simulink model "planarModel"  (R2018b)
settings: Solver=FixedStepAuto  StartTime=0.0  StopTime=50  FixedStep=0.025  RelTol=1e-3
InitFcn:
  | loadThrusterData
settings Model: Creator=Andy  LastModifiedBy=barthal
settings ModelReferenceCC: ModelReferenceNumInstancesAllowed=Single
settings RTWCC: GenCodeOnly=on

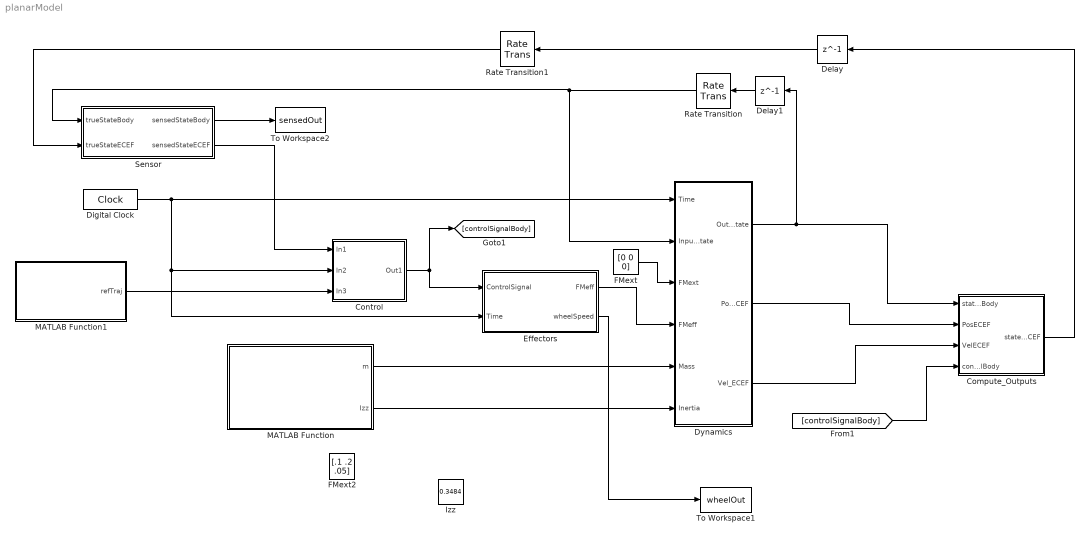
== system planarModel ==
  Compute_Outputs : Subsystem
  Control : Subsystem
  Delay : Delay  DelayLength=1
  Delay1 : Delay  DelayLength=1
  Digital Clock : DigitalClock  SampleTime=0.025
  Dynamics : Subsystem  TreatAsAtomicUnit=on
      settings: MinAlgLoopOccurrences=on
  Effectors : Subsystem  TreatAsAtomicUnit=on
  FMext : Constant  Value=[0 0 0]
  FMext2 : Constant  Value=[.1 .2 .05]
  Izz : Constant  Value=0.3484
  MATLAB Function : MATLAB Function  TreatAsAtomicUnit=on
  MATLAB Function1 : MATLAB Function  TreatAsAtomicUnit=on
  Rate Transition : RateTransition  InitialCondition=[0 0 0 0 0 0 0 0 0]
  Rate Transition1 : RateTransition  InitialCondition=[0 0 0 0 0 0 0 0 0]
  Sensor : Subsystem
  To Workspace1 : ToWorkspace  VariableName=wheelOut  SaveFormat=Timeseries  SampleTime=-1
  To Workspace2 : ToWorkspace  VariableName=sensedOut  SaveFormat=Timeseries  SampleTime=-1
  wires:
  Digital Clock/1 -> Dynamics/1(Time), Control/2(In2), Effectors/2(Time)
  FMext/1 -> Dynamics/3(FMext)
  MATLAB Function/1(m) -> Dynamics/5(Mass)
  Effectors/2(wheelSpeed) -> To Workspace1/1
  Control/1(Out1) -> [controlSignalBody], Effectors/1(ControlSignal)
  Effectors/1(FMeff) -> Dynamics/4(FMeff)
  Dynamics/1(OutputState) -> Delay1/1, Compute_Outputs/1(stateInBody)
  Dynamics/2(Pos_ECEF) -> Compute_Outputs/2(PosECEF)
  Dynamics/3(Vel_ECEF) -> Compute_Outputs/3(VelECEF)
  Compute_Outputs/1(stateOutECEF) -> Delay/1
  [controlSignalBody] -> Compute_Outputs/4(controlSignalBody)
  MATLAB Function/2(Izz) -> Dynamics/6(Inertia)
  Rate Transition/1 -> Sensor/1(trueStateBody), Dynamics/2(InputState)
  Rate Transition1/1 -> Sensor/2(trueStateECEF)
  Sensor/2(sensedStateECEF) -> Control/1(In1)
  Sensor/1(sensedStateBody) -> To Workspace2/1
  MATLAB Function1/1(refTraj) -> Control/3(In3)
  Delay/1 -> Rate Transition1/1
  Delay1/1 -> Rate Transition/1

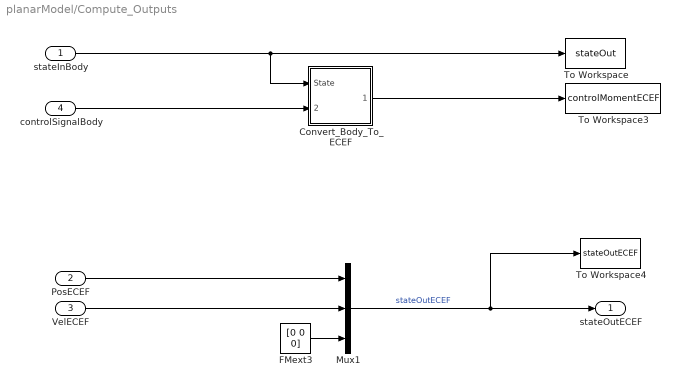
== system planarModel/Compute_Outputs ==
  stateInBody : Inport
  PosECEF : Inport  Port=2
  VelECEF : Inport  Port=3
  controlSignalBody : Inport  Port=4
  Convert_Body_To_ECEF : Subsystem
  FMext3 : Constant  Value=[0 0 0]
  Mux1 : Mux  Inputs=3
  To Workspace : ToWorkspace  VariableName=stateOut  SaveFormat=Timeseries  SampleTime=-1
  To Workspace3 : ToWorkspace  VariableName=controlMomentECEF  SaveFormat=Timeseries  SampleTime=-1
  To Workspace4 : ToWorkspace  VariableName=stateOutECEF  SaveFormat=Timeseries  SampleTime=-1
  stateOutECEF : Outport
  wires:
  Mux1/1 -> stateOutECEF/1, To Workspace4/1  "stateOutECEF"
  FMext3/1 -> Mux1/3
  stateInBody/1 -> Convert_Body_To_ECEF/1(State), To Workspace/1
  Convert_Body_To_ECEF/1(Vec_ECEF) -> To Workspace3/1
  controlSignalBody/1 -> Convert_Body_To_ECEF/2(Vec_Body)
  PosECEF/1 -> Mux1/1
  VelECEF/1 -> Mux1/2

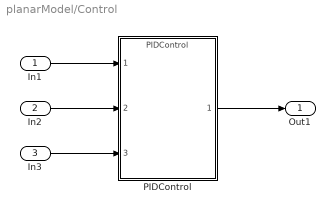
== system planarModel/Control ==
  In1 : Inport
  In2 : Inport  Port=2
  In3 : Inport  Port=3
  PIDControl : ModelReference  ModelNameDialog=PIDControl  SimulationMode=Normal  ModelReferenceVersion=1.303
  Out1 : Outport
  wires:
  In3/1 -> PIDControl/3
  In2/1 -> PIDControl/2
  PIDControl/1 -> Out1/1
  In1/1 -> PIDControl/1

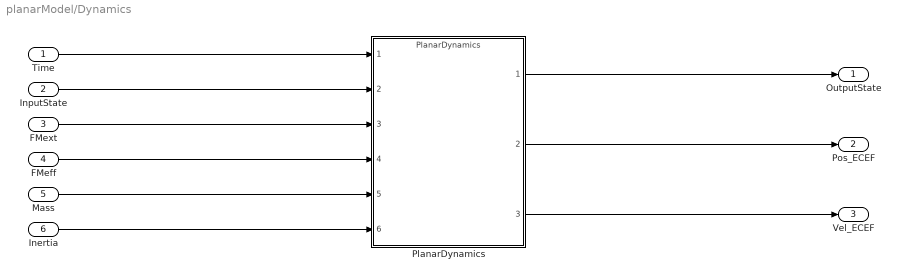
== system planarModel/Dynamics ==
  Time : Inport
  InputState : Inport  Port=2
  FMext : Inport  Port=3
  FMeff : Inport  Port=4
  Mass : Inport  Port=5
  Inertia : Inport  Port=6
  PlanarDynamics : ModelReference  ModelNameDialog=PlanarDynamics  SimulationMode=Normal  ModelReferenceVersion=1.307
  OutputState : Outport
  Pos_ECEF : Outport  Port=2
  Vel_ECEF : Outport  Port=3
  wires:
  Time/1 -> PlanarDynamics/1
  InputState/1 -> PlanarDynamics/2
  FMext/1 -> PlanarDynamics/3
  FMeff/1 -> PlanarDynamics/4
  Mass/1 -> PlanarDynamics/5
  Inertia/1 -> PlanarDynamics/6
  PlanarDynamics/1 -> OutputState/1
  PlanarDynamics/2 -> Pos_ECEF/1
  PlanarDynamics/3 -> Vel_ECEF/1

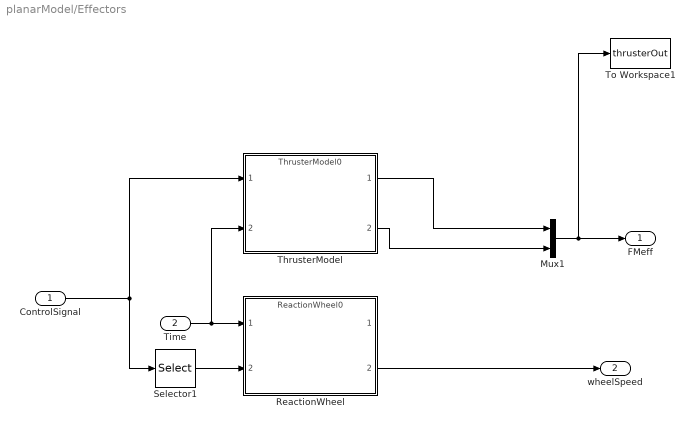
== system planarModel/Effectors ==
  ControlSignal : Inport
  Time : Inport  Port=2
  Mux1 : Mux  Inputs=2
  ReactionWheel : ModelReference  ModelNameDialog=ReactionWheel0  SimulationMode=Normal  ModelReferenceVersion=1.301
  Selector1 : Selector  InputPortWidth=3  IndexOptions=Index vector (dialog)  Indices=[3]  OutputSizes=1
  ThrusterModel : ModelReference  ModelNameDialog=ThrusterModel0  SimulationMode=Normal  ModelReferenceVersion=1.301
  To Workspace1 : ToWorkspace  VariableName=thrusterOut  SaveFormat=Timeseries  SampleTime=-1
  FMeff : Outport
  wheelSpeed : Outport  Port=2
  wires:
  Mux1/1 -> FMeff/1, To Workspace1/1
  Selector1/1 -> ReactionWheel/2
  ReactionWheel/2 -> wheelSpeed/1
  ControlSignal/1 -> ThrusterModel/1, Selector1/1
  Time/1 -> ThrusterModel/2, ReactionWheel/1
  ThrusterModel/1 -> Mux1/1
  ThrusterModel/2 -> Mux1/2

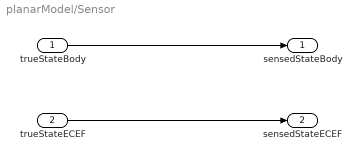
== system planarModel/Sensor ==
  trueStateBody : Inport  OutDataTypeStr=double  PortDimensions=9  SampleTime=[0.025000000000000001,0]
  trueStateECEF : Inport  Port=2  OutDataTypeStr=double  PortDimensions=9  SampleTime=[0.025000000000000001,0]
  sensedStateBody : Outport  OutDataTypeStr=double  PortDimensions=9  SampleTime=[0.025000000000000001,0]
  sensedStateECEF : Outport  Port=2  OutDataTypeStr=double  PortDimensions=9  SampleTime=[0.025000000000000001,0]
  wires:
  trueStateBody/1 -> sensedStateBody/1
  trueStateECEF/1 -> sensedStateECEF/1

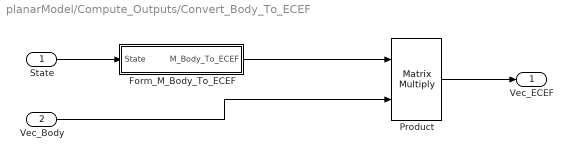
== system planarModel/Compute_Outputs/Convert_Body_To_ECEF ==
  State : Inport  PortDimensions=9
  Vec_Body : Inport  Port=2  PortDimensions=3
  Form_M_Body_To_ECEF : Subsystem
  Product : Product  Multiplication=Matrix(*)
  Vec_ECEF : Outport  PortDimensions=3
  wires:
  State/1 -> Form_M_Body_To_ECEF/1(State)
  Form_M_Body_To_ECEF/1(M_Body_To_ECEF) -> Product/1
  Vec_Body/1 -> Product/2
  Product/1 -> Vec_ECEF/1

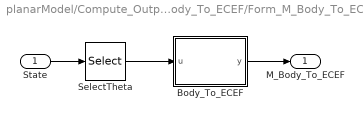
== system planarModel/Compute_Outputs/Convert_Body_To_ECEF/Form_M_Body_To_ECEF ==
  State : Inport
  Body_To_ECEF : MATLAB Function  TreatAsAtomicUnit=on
  SelectTheta : Selector  InputPortWidth=9  IndexOptions=Index vector (dialog)  Indices=3  OutputSizes=1
  M_Body_To_ECEF : Outport
  wires:
  State/1 -> SelectTheta/1
  SelectTheta/1 -> Body_To_ECEF/1(u)
  Body_To_ECEF/1(y) -> M_Body_To_ECEF/1

== matlab function planarModel/MATLAB Function ==
  data: m output; Izz output
function [m,Izz] = callplanarMassProperties

[m Izz] = planarMassProperties();

== matlab function planarModel/Compute_Outputs/Convert_Body_To_ECEF/Form_M_Body_To_ECEF/Body_To_ECEF ==
  data: u input; y output
function y = fcn(u)

y = [cos(u) -sin(u) 0; sin(u) cos(u) 0;0 0 1];

== matlab function planarModel/MATLAB Function1 ==
  data: refTraj output
function refTraj  = callreferenceTrajectory

[refTraj] = referenceTrajectory();
